simulink model "HDLDownshifter"  (R2024a)
settings: Solver=FixedStepDiscrete  StartTime=0.0  StopTime=stopTime  RelTol=1e-3
undefined symbols (not defined in the file or in its folder): CONST
libraries: dspsrcs4 x3, HDL_ieee_8021513 x2, whdlutilities x1
settings Model: DataTypeOverride=Off  Creator=cotti  LastModifiedBy=cotti
settings OptimizationCC: BlockReduction=off  ConditionallyExecuteInputs=off  DefaultParameterBehavior=Inlined  InheritOutputTypeSmallerThanSingle=on
settings DebuggingCC: AlgebraicLoopMsg=error  ArtificialAlgebraicLoopMsg=error  SingleTaskRateTransMsg=error  UnconnectedInputMsg=warning  UnconnectedOutputMsg=warning  UnconnectedLineMsg=warning
settings HardwareCC: ProdBitPerPointer=32  ProdBitPerSizeT=32  ProdBitPerPtrDiffT=32  ProdLargestAtomicFloat=None  ProdIntDivRoundTo=Undefined  ProdEndianess=Unspecified  ProdWordSize=32  ProdHWDeviceType=ASIC/FPGA->ASIC/FPGA  TargetBitPerLong=64  TargetBitPerPointer=64  TargetBitPerSizeT=64  TargetBitPerPtrDiffT=64  TargetLongLongMode=on  TargetIntDivRoundTo=Zero  TargetEndianess=LittleEndian  TargetWordSize=64  TargetHWDeviceType=Custom Processor->MATLAB Host Computer  ProdEqTarget=off

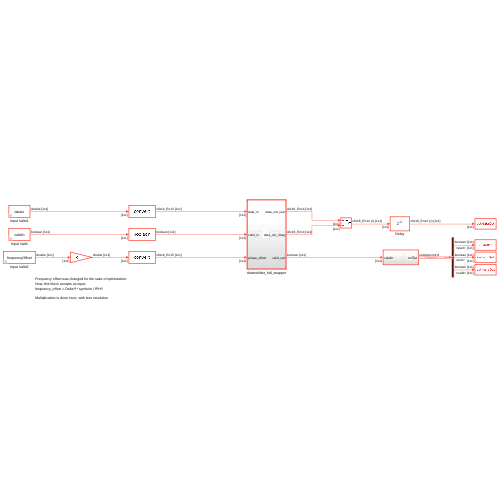
[thumbnail: Simulink's stored preview of the top-level diagram]
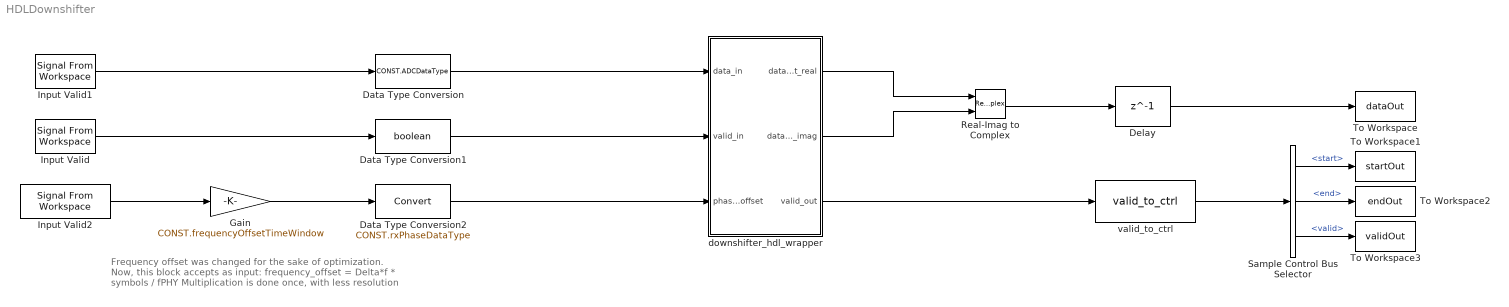
== system HDLDownshifter ==
  note: Frequency offset was changed for the sake of optimization.
      | Now, this block accepts as input:
      | frequency_offset = Delta*f * symbols / fPHY
      |
      | Multiplication is done once, with less resolution
  Data Type Conversion : DataTypeConversion  OutDataTypeStr=CONST.ADCDataType  SaturateOnIntegerOverflow=off  RndMeth=Floor
  Data Type Conversion1 : DataTypeConversion  OutDataTypeStr=boolean  SaturateOnIntegerOverflow=off  RndMeth=Floor
  Data Type Conversion2 : DataTypeConversion  OutDataTypeStr=CONST.rxPhaseDataType  SaturateOnIntegerOverflow=off  RndMeth=Floor
  Delay : Delay  DelayLength=1  InitialCondition=0  UseCircularBuffer=on
  Gain : Gain  Gain=CONST.frequencyOffsetTimeWindow
  Input Valid : dspsrcs4/Signal From Workspace  X=validIn  Ts=1/CONST.fADC  nsamps=1  OutputAfterFinalValue=Setting to zero  ignoreOrWarnInputAndFrameLengths=off  OutputFrames=off
  Input Valid1 : dspsrcs4/Signal From Workspace  X=dataIn  Ts=1/CONST.fADC  nsamps=1  OutputAfterFinalValue=Setting to zero  ignoreOrWarnInputAndFrameLengths=off  OutputFrames=off
  Input Valid2 : dspsrcs4/Signal From Workspace  X=frequencyOffset  Ts=1/CONST.fADC  nsamps=1  OutputAfterFinalValue=Setting to zero  ignoreOrWarnInputAndFrameLengths=off  OutputFrames=off
  Real-Imag to Complex : RealImagToComplex
  Sample Control Bus Selector : whdlutilities/Sample Control Bus Selector  OutputSignals=start,end,valid
  To Workspace : ToWorkspace  VariableName=dataOut  SampleTime=1/CONST.fADC
      settings: Save2DSignal=2-D array (concatenate along first dimension)
  To Workspace1 : ToWorkspace  VariableName=startOut  SampleTime=1/CONST.fADC
      settings: Save2DSignal=2-D array (concatenate along first dimension)
  To Workspace2 : ToWorkspace  VariableName=endOut  SampleTime=1/CONST.fADC
      settings: Save2DSignal=2-D array (concatenate along first dimension)
  To Workspace3 : ToWorkspace  VariableName=validOut  SampleTime=1/CONST.fADC
      settings: Save2DSignal=2-D array (concatenate along first dimension)
  downshifter_hdl_wrapper : Subsystem  TreatAsAtomicUnit=on
  valid_to_ctrl : HDL_ieee_8021513/valid_to_ctrl  SystemSampleTime=-1  VariantActivationTime=update diagram  AllowFlexibleInterface=on  Latency=0  AutoFrameSizeCalculation=off
      settings: SourceProductName=HDL IEEE 8021513
  wires:
  Input Valid/1 -> Data Type Conversion1/1
  Input Valid1/1 -> Data Type Conversion/1
  Sample Control Bus Selector/2 -> To Workspace2/1  "<end>"
  valid_to_ctrl/1 -> Sample Control Bus Selector/1
  Sample Control Bus Selector/1 -> To Workspace1/1  "<start>"
  Sample Control Bus Selector/3 -> To Workspace3/1  "<valid>"
  Delay/1 -> To Workspace/1
  Input Valid2/1 -> Gain/1
  Gain/1 -> Data Type Conversion2/1
  Data Type Conversion/1 -> downshifter_hdl_wrapper/1(data_in)
  Data Type Conversion1/1 -> downshifter_hdl_wrapper/2(valid_in)
  Data Type Conversion2/1 -> downshifter_hdl_wrapper/3(phase_offset)
  downshifter_hdl_wrapper/3(valid_out) -> valid_to_ctrl/1
  Real-Imag to Complex/1 -> Delay/1
  downshifter_hdl_wrapper/1(data_out_real) -> Real-Imag to Complex/1
  downshifter_hdl_wrapper/2(data_out_imag) -> Real-Imag to Complex/2

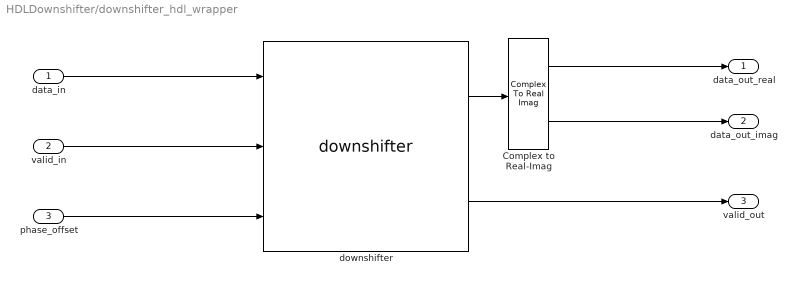
== system HDLDownshifter/downshifter_hdl_wrapper ==
  data_in : Inport
  valid_in : Inport  Port=2
  phase_offset : Inport  Port=3
  Complex to Real-Imag : ComplexToRealImag
  downshifter : HDL_ieee_8021513/downshifter  SystemSampleTime=-1  VariantActivationTime=update diagram  AllowFlexibleInterface=on  Latency=0  AutoFrameSizeCalculation=off
      settings: SourceProductName=HDL IEEE 8021513
  data_out_real : Outport
  data_out_imag : Outport  Port=2
  valid_out : Outport  Port=3
  wires:
  downshifter/1 -> Complex to Real-Imag/1
  Complex to Real-Imag/2 -> data_out_imag/1
  Complex to Real-Imag/1 -> data_out_real/1
  downshifter/2 -> valid_out/1
  data_in/1 -> downshifter/1
  valid_in/1 -> downshifter/2
  phase_offset/1 -> downshifter/3
